simulink model "J2_drag"  (R2020b)
settings: Solver=VariableStepAuto  StartTime=0.0  StopTime=T  RelTol=1e-3
model workspace (MAT data in the model file):
  y_0 = 0
values from neighbouring files (symbols this model uses):
  Cd = 2.0    (= 2)    [main_old.m]    (also in mon_main.m = 2.2; orbit.m = 2.2; setup.m)
  rho = 42.418*10^-11    (= 4.2418e-10)    [main_old.m]    (also in mon_main.m = 2.6e-12; orbit.m = 2.6e-12; setup.m)
  S = create_spacecraft(center, R, dim)    [anim_old.m]    (also in mon_main.m = 0.01; orbit.m = 0.01; start_anim_old.m = create_spacecraft(center, Rib, dim); start_animation_old.m = Ss(:,3*k-2:3*k))
settings Model: Creator=djoff  LastModifiedBy=djoff

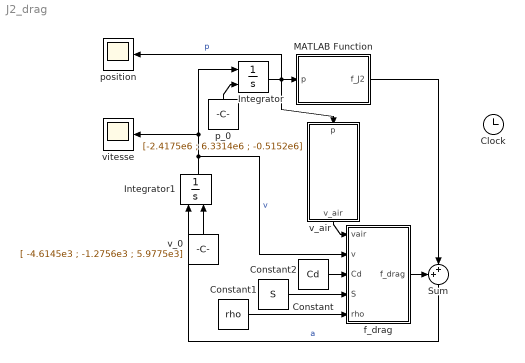
== system J2_drag ==
  Clock : Clock
  Constant : Constant  Value=Cd
  Constant1 : Constant  Value=rho
  Constant2 : Constant  Value=S
  Integrator : Integrator  InitialConditionSource=external
  Integrator1 : Integrator  InitialConditionSource=external
  MATLAB Function : MATLAB Function  TreatAsAtomicUnit=on
  Sum : Sum  Inputs=++|
  f_drag : MATLAB Function  TreatAsAtomicUnit=on
  p_0 : Constant  Value=[-2.4175e6 ; 6.3314e6 ; -0.5152e6]
  position : Scope
  v_0 : Constant  Value=[ -4.6145e3 ; -1.2756e3 ; 5.9775e3]
  v_air : MATLAB Function  TreatAsAtomicUnit=on
  vitesse : Scope
  wires:
  v_air/1(v_air) -> f_drag/1(vair)
  Integrator/1 -> position/1, v_air/1(p), MATLAB Function/1(p)  "p"
  p_0/1 -> Integrator/2
  Integrator1/1 -> Integrator/1, vitesse/1, f_drag/2(v)  "v"
  v_0/1 -> Integrator1/2
  f_drag/1(f_drag) -> Sum/1
  MATLAB Function/1(f_J2) -> Sum/2
  Sum/1 -> Integrator1/1  "a"
  Constant/1 -> f_drag/3(Cd)
  Constant2/1 -> f_drag/4(S)
  Constant1/1 -> f_drag/5(rho)

== matlab function J2_drag/f_drag ==
  data: vair input; v input; f_drag output; Cd input; S input; rho input
function f_drag = f_drag(vair,v,Cd,S,rho)

fdrag(4:6)=-1/2*Cd*S*rho*(norm(v-vair))*(v-vair);
end

== matlab function J2_drag/v_air ==
  data: v_air output; p input
function v_air = v_air(p)
r=norm(p);
co=p(2)/sqrt(p(1)^2+p(2)^2);
si=p(1)/sqrt(p(1)^2+p(2)^2);
colambda=sqrt(p(1)^2+p(2)^2)/r;
v_air=2*pi/(24*3600)*r*colambda*[-si co 0];
end

== matlab function J2_drag/MATLAB Function ==
  data: p input; f_J2 output
function f_J2 = J2(p)
r=norm(p)

f_J2(1) = -mu/r^3*p(1) -3/2*J2*(mu/r^2)*(Re/r)^2*(1-5*(p(3)/r)^2)*p(1)/r;
f_J2(2) = -mu/r^3*p(2) -3/2*J2*(mu/r^2)*(Re/r)^2*(1-5*(p(3)/r)^2)*p(2)/r;
f_J2(3) = -mu/r^3*p(3) -3/2*J2*(mu/r^2)*(Re/r)^2*(3-5*(p(3)/r)^2)*p(3)/r;
end
